simulink subsystem "BMS"  (R2019b)
settings: Solver=VariableStepAuto  StartTime=0.0  StopTime=10.0  RelTol=1e-3
undefined symbols (not defined in the file or in its folder): C1_lut, C2_lut, OCV_lut, R0_est, R0_lut, R2_lut
libraries: sharedTrackingLibrary x1
settings Model: Creator=PcElettronicaDynamis  LastModifiedBy=PcElettronicaDynamis

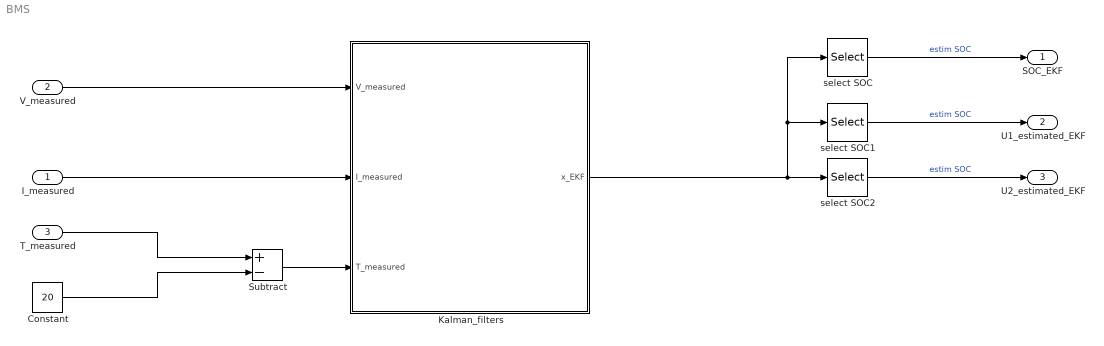
== system BMS ==
  I_measured : Inport
  V_measured : Inport  Port=2
  T_measured : Inport  Port=3
  Constant : Constant  Value=20
  Kalman_filters : Subsystem
  Subtract : Sum  Inputs=+-
  select SOC : Selector  InputPortWidth=3  IndexOptions=Index vector (dialog)  Indices=1  OutputSizes=1
  select SOC1 : Selector  InputPortWidth=3  IndexOptions=Index vector (dialog)  Indices=2  OutputSizes=1
  select SOC2 : Selector  InputPortWidth=3  IndexOptions=Index vector (dialog)  Indices=3  OutputSizes=1
  SOC_EKF : Outport
  U1_estimated_EKF : Outport  Port=2
  U2_estimated_EKF : Outport  Port=3
  wires:
  Kalman_filters/1(x_EKF) -> select SOC2/1, select SOC1/1, select SOC/1
  select SOC2/1 -> U2_estimated_EKF/1  "estim SOC"
  Constant/1 -> Subtract/2
  Subtract/1 -> Kalman_filters/3(T_measured)
  I_measured/1 -> Kalman_filters/2(I_measured)
  T_measured/1 -> Subtract/1
  select SOC1/1 -> U1_estimated_EKF/1  "estim SOC"
  select SOC/1 -> SOC_EKF/1  "estim SOC"
  V_measured/1 -> Kalman_filters/1(V_measured)

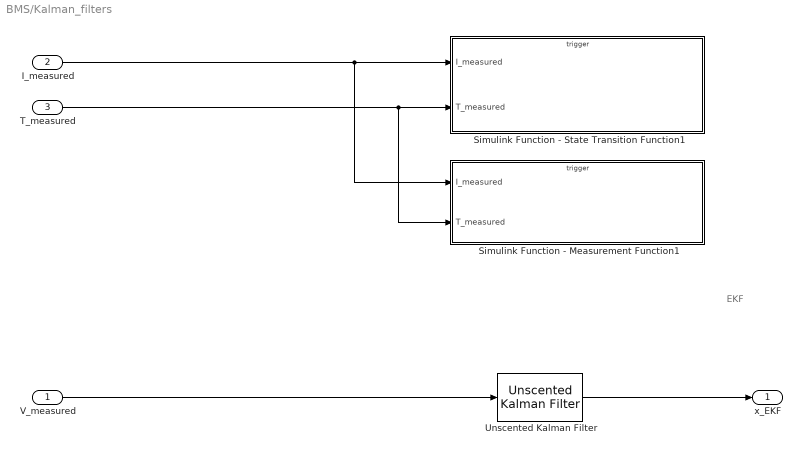
== system BMS/Kalman_filters ==
  note: EKF
  V_measured : Inport
  I_measured : Inport  Port=2
  T_measured : Inport  Port=3
  Simulink Function - Measurement Function1 : Subsystem  TreatAsAtomicUnit=on
  Simulink Function - State Transition Function1 : Subsystem  TreatAsAtomicUnit=on
  Unscented Kalman Filter : sharedTrackingLibrary/Unscented Kalman Filter  StateTransitionFcn=batteryStateFcn_UKF  HasAdditiveProcessNoise=Additive  ProcessNoise=diag([1e-12, 1e-12, 1e-12])  HasTimeVaryingProcessNoise=off  HasStateTransitionFcnExtraArgument=0  InitialState=[0.2,0,0]  InitialStateCovariance=diag([0.5,0.001,0.001])  Alpha=1e-3  Beta=2  Kappa=0  MeasurementFcn1=batteryMeasurementFcn_UKF  HasMeasurementEnablePort1=off  HasAdditiveMeasurementNoise1=Additive  MeasurementNoise1=1  HasTimeVaryingMeasurementNoise1=off  HasMeasurementFcnExtraArgument1=0  MeasurementFcn2=myMeasurementFcn  HasMeasurementEnablePort2=off  HasAdditiveMeasurementNoise2=Additive  MeasurementNoise2=1  HasTimeVaryingMeasurementNoise2=off  HasMeasurementFcnExtraArgument2=0  MeasurementFcn3=myMeasurementFcn  HasMeasurementEnablePort3=off  HasAdditiveMeasurementNoise3=Additive  MeasurementNoise3=1  HasTimeVaryingMeasurementNoise3=off  HasMeasurementFcnExtraArgument3=0  MeasurementFcn4=myMeasurementFcn  HasMeasurementEnablePort4=off  HasAdditiveMeasurementNoise4=Additive  MeasurementNoise4=1  HasTimeVaryingMeasurementNoise4=off  HasMeasurementFcnExtraArgument4=0  MeasurementFcn5=myMeasurementFcn  HasMeasurementEnablePort5=off  HasAdditiveMeasurementNoise5=Additive  MeasurementNoise5=1  HasTimeVaryingMeasurementNoise5=off  HasMeasurementFcnExtraArgument5=0  EnableMultirate=off  StateTransitionFcnSampleTime=1  MeasurementFcn1SampleTime=1  MeasurementFcn2SampleTime=1  MeasurementFcn3SampleTime=1  MeasurementFcn4SampleTime=1  MeasurementFcn5SampleTime=1  UseCurrentEstimator=on  OutputStateCovariance=off  DataType=double  SampleTime=0.1  NumberOfMeasurements=1
      settings: SourceProductName=Automated Driving Toolbox  SourceProductBaseCode=DR
  x_EKF : Outport  VectorParamsAs1DForOutWhenUnconnected=off
  wires:
  Unscented Kalman Filter/1 -> x_EKF/1
  T_measured/1 -> Simulink Function - State Transition Function1/2(T_measured), Simulink Function - Measurement Function1/2(T_measured)
  I_measured/1 -> Simulink Function - State Transition Function1/1(I_measured), Simulink Function - Measurement Function1/1(I_measured)
  V_measured/1 -> Unscented Kalman Filter/1

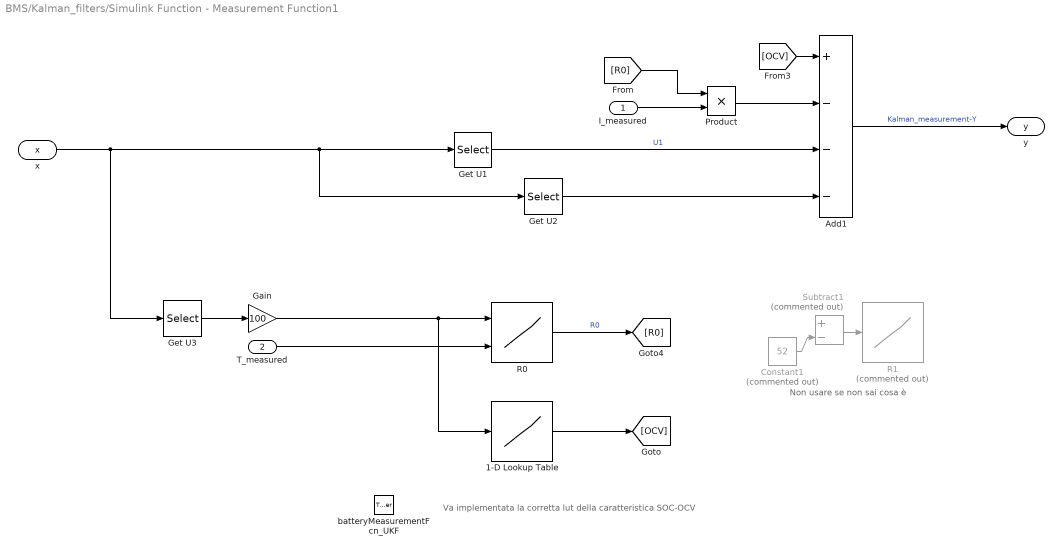
== system BMS/Kalman_filters/Simulink Function - Measurement Function1 ==
  note: Va implementata la corretta lut della caratteristica SOC-OCV
  note: Non usare se non sai cosa è
  I_measured : Inport
  T_measured : Inport  Port=2
  batteryMeasurementFcn_UKF : TriggerPort  TriggerType=function-call  IsSimulinkFunction=on  FunctionName=batteryMeasurementFcn_UKF  VariantControl=Variant
  1-D Lookup Table : Lookup_n-D  NumberOfTableDimensions=1  BreakpointsForDimension1=[1:100]  BreakpointsForDimension2=[1:40]  BreakpointsForDimension1FirstPoint=0  BreakpointsForDimension1Spacing=10  Table=OCV_lut  InternalRulePriority=Speed  RndMeth=Simplest  InputSameDT=on
  Add1 : Sum  Inputs=+---
  Constant1 : Constant  Commented=on  Value=52
  Gain : Gain  Gain=100
  Get U1 : Selector  InputPortWidth=3  IndexOptions=Index vector (dialog)  Indices=2  OutputSizes=1
  Get U2 : Selector  InputPortWidth=3  IndexOptions=Index vector (dialog)  Indices=3  OutputSizes=1
  Get U3 : Selector  InputPortWidth=3  IndexOptions=Index vector (dialog)  Indices=1  OutputSizes=1
  Product : Product
  R0 : Lookup_n-D  BreakpointsForDimension1=[1:100]  BreakpointsForDimension2=[1:40]  BreakpointsForDimension1FirstPoint=0  BreakpointsForDimension1Spacing=10  Table=R0_lut  InternalRulePriority=Speed  RndMeth=Simplest  InputSameDT=on
  R1 : Lookup_n-D  Commented=on  NumberOfTableDimensions=1  BreakpointsForDimension1=[1:32]  BreakpointsForDimension2=[1:40]  BreakpointsForDimension1FirstPoint=0  BreakpointsForDimension1Spacing=10  Table=R0_est  InternalRulePriority=Speed  RndMeth=Simplest  InputSameDT=on
  Subtract1 : Sum  Commented=on  Inputs=+-
  x : ArgIn  DisableCoverage=on  PortDimensions=3  ArgumentName=x
  y : ArgOut  DisableCoverage=on  ArgumentName=y
  wires:
  Constant1/1 -> Subtract1/2
  Subtract1/1 -> R1/1
  Gain/1 -> 1-D Lookup Table/1, R0/1
  1-D Lookup Table/1 -> [OCV]
  [OCV] -> Add1/1
  Get U3/1 -> Gain/1
  I_measured/1 -> Product/2
  [R0] -> Product/1
  T_measured/1 -> R0/2
  R0/1 -> [R0]  "R0"
  Get U2/1 -> Add1/4
  Get U1/1 -> Add1/3  "U1"
  Product/1 -> Add1/2
  Add1/1 -> y/1  "Kalman_measurement-Y"
  x/1 -> Get U1/1, Get U2/1, Get U3/1

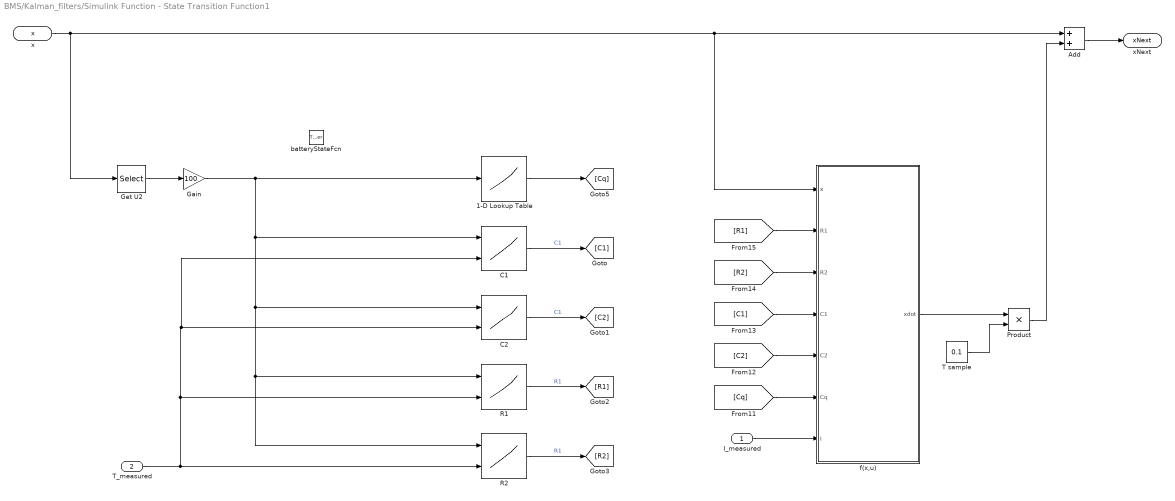
== system BMS/Kalman_filters/Simulink Function - State Transition Function1 ==
  I_measured : Inport
  T_measured : Inport  Port=2
  batteryStateFcn : TriggerPort  TriggerType=function-call  IsSimulinkFunction=on  FunctionName=batteryStateFcn_UKF  VariantControl=Variant
  1-D Lookup Table : Lookup_n-D  NumberOfTableDimensions=1  BreakpointsForDimension1=1:10:100  Table=[3.2 3.2 3.2 3.2 3.2 3.2 3.2 3.2 3.2 3.2]  InternalRulePriority=Speed  RndMeth=Simplest  InputSameDT=on
  Add : Sum
  C1 : Lookup_n-D  BreakpointsForDimension1=[1:100]  BreakpointsForDimension2=[1:40]  BreakpointsForDimension1FirstPoint=0  BreakpointsForDimension1Spacing=10  Table=C1_lut  InternalRulePriority=Speed  RndMeth=Simplest  InputSameDT=on
  C2 : Lookup_n-D  BreakpointsForDimension1=[1:100]  BreakpointsForDimension2=[1:40]  BreakpointsForDimension1FirstPoint=0  BreakpointsForDimension1Spacing=10  Table=C2_lut  InternalRulePriority=Speed  RndMeth=Simplest  InputSameDT=on
  Gain : Gain  Gain=100
  Get U2 : Selector  InputPortWidth=3  IndexOptions=Index vector (dialog)  Indices=1  OutputSizes=1
  Product : Product
  R1 : Lookup_n-D  BreakpointsForDimension1=[1:100]  BreakpointsForDimension2=[1:40]  BreakpointsForDimension1FirstPoint=0  BreakpointsForDimension1Spacing=10  Table=R0_lut  InternalRulePriority=Speed  RndMeth=Simplest  InputSameDT=on
  R2 : Lookup_n-D  BreakpointsForDimension1=[1:100]  BreakpointsForDimension2=[1:40]  BreakpointsForDimension1FirstPoint=0  BreakpointsForDimension1Spacing=10  Table=R2_lut  InternalRulePriority=Speed  RndMeth=Simplest  InputSameDT=on
  T sample : Constant  Value=0.1
  f(x,u) : MATLAB Function  TreatAsAtomicUnit=on
  x : ArgIn  DisableCoverage=on  PortDimensions=3  ArgumentName=x
  xNext : ArgOut  DisableCoverage=on  PortDimensions=3  ArgumentName=xNext
  wires:
  Gain/1 -> C1/1, C2/1, R1/1, R2/1, 1-D Lookup Table/1
  1-D Lookup Table/1 -> [Cq]
  Get U2/1 -> Gain/1
  I_measured/1 -> f(x,u)/7(I)
  [Cq] -> f(x,u)/6(Cq)
  [C2] -> f(x,u)/5(C2)
  [C1] -> f(x,u)/4(C1)
  [R2] -> f(x,u)/3(R2)
  [R1] -> f(x,u)/2(R1)
  T_measured/1 -> R2/2, R1/2, C2/2, C1/2
  C2/1 -> [C2]  "C1"
  C1/1 -> [C1]  "C1"
  R2/1 -> [R2]  "R1"
  R1/1 -> [R1]  "R1"
  Product/1 -> Add/2
  f(x,u)/1(xdot) -> Product/1
  T sample/1 -> Product/2
  Add/1 -> xNext/1
  x/1 -> Get U2/1, f(x,u)/1(x), Add/1

== matlab function BMS/Kalman_filters/Simulink Function - State Transition Function1/f(x,u) ==
  data: x input; R1 input; R2 input; C1 input; C2 input; Cq input; I input; xdot output
function xdot = fx(x,R1,R2,C1,C2,Cq,I)

t1 = C1*R1;
t2 = C2*R2;

xdot = zeros(size(x));

U1 = x(2);
U2 = x(3);

xdot(1) =  -I/(3600*Cq);
xdot(2) = -(1/t1)*U1 + I/(t1/R1);
xdot(3) = -(1/t2)*U2 + I/(t2/R2);
